simulink model "S_PIL_PVSISTEM_2026_V1"  (R2017a)
settings: Solver=VariableStepAuto  StartTime=0.0  StopTime=1.3  FixedStep=1e-6  MaxStep=1e-4  RelTol=1e-3
values from neighbouring files (symbols this model uses):
  a = 9    [M_PARAM_V1.m]    (also in M_PIL_PVSISTEM_2026_V1.m; ModTusk_V1.m)
  Alpha1 = 2*Zeta_obs*wn_obs    (= 2)    [M_PARAM_V1.m]    (also in M_PIL_PVSISTEM_2026_V1.m)
  Alpha2 = wn_obs    (= 1)    [M_PARAM_V1.m]    (also in M_PIL_PVSISTEM_2026_V1.m)
  alpha_max = 4/ts_min    (= 13333.3333333)    [M_PARAM_V1.m]    (also in M_PIL_PVSISTEM_2026_V1.m; ModTusk_V1.m)
  alpha_min = 4/ts_max    (= 259.067357513)    [M_PARAM_V1.m]    (also in M_PIL_PVSISTEM_2026_V1.m = 133.333333333; ModTusk_V1.m = 133.333333333)
  Cdc = Cdc    (= 0.0033)    [M_PARAM_V1.m]    (also in M_PIL_PVSISTEM_2026_V1.m = 0.00047)
  Cpv = Cpv    (= 0.0001)    [M_PARAM_V1.m]    (also in M_PIL_PVSISTEM_2026_V1.m = 0.0002)
  dIL = (vpv/L)*d*Ts    (= 0.46035072)    [M_PIL_PVSISTEM_2026_V1.m]
  Epsilon = Ep_cont/Ts1    [M_PARAM_V1.m]    (also in M_PIL_PVSISTEM_2026_V1.m)
  ESRCdc = ESRCdc    (= 0.2)    [M_PARAM_V1.m]    (also in M_PIL_PVSISTEM_2026_V1.m)
  ESRCpv = ESRCpv    (= 0.2)    [M_PARAM_V1.m]    (also in M_PIL_PVSISTEM_2026_V1.m)
  Fred = fs    (= 60)    [M_PARAM_V1.m]    (also in M_PIL_PVSISTEM_2026_V1.m)
  fs = 60    [M_PARAM_V1.m]    (also in M_PIL_PVSISTEM_2026_V1.m)
  Icc_calc = In/(5/100)    [M_PARAM_V1.m]    (also in M_PIL_PVSISTEM_2026_V1.m)
  K1 = Kt_acker_d    [M_PARAM_V1.m]    (also in M_PIL_PVSISTEM_2026_V1.m)
  K1y2md = Kmd(1:end-1)    [M_PARAM_V1.m]    (also in M_PIL_PVSISTEM_2026_V1.m)
  Kdpwm = 1/Ucmax    (= 0.000111111111111)    [M_PARAM_V1.m]    (also in M_PIL_PVSISTEM_2026_V1.m = 1.52590218967e-05)
  KI1 = Kp1/Ti1*Ts1    (= 760)    [M_PARAM_V1.m]    (also in M_PIL_PVSISTEM_2026_V1.m = 14.4)
  KI2 = Ki2*Ts4    [M_PARAM_V1.m]    (also in M_PIL_PVSISTEM_2026_V1.m)
  KI4 = Ki4*Ts4    [M_PARAM_V1.m]    (also in M_PIL_PVSISTEM_2026_V1.m)
  KI5 = Ki5*Ts_inv    (= 0.17765287922)    [M_PARAM_V1.m]    (also in M_PIL_PVSISTEM_2026_V1.m = 0.0710611516878)
  Kimd = -Kmd(end)    [M_PARAM_V1.m]    (also in M_PIL_PVSISTEM_2026_V1.m)
  KP1 = Kp1-KI1/2    (= 5320)    [M_PARAM_V1.m]    (also in M_PIL_PVSISTEM_2026_V1.m = 2392.8)
  KP2 = Kp2-KI2/2    [M_PARAM_V1.m]    (also in M_PIL_PVSISTEM_2026_V1.m)
  KP4 = Kp4-KI4/2    [M_PARAM_V1.m]    (also in M_PIL_PVSISTEM_2026_V1.m)
  KP5 = Kp5*Ts_inv-KI5/2    (= -0.0874937760062)    [M_PARAM_V1.m]    (also in M_PIL_PVSISTEM_2026_V1.m = -0.0349975104025)
  L = L    (= 0.0044)    [M_PARAM_V1.m]    (also in M_PIL_PVSISTEM_2026_V1.m = 0.1)
  Linv = 0.03    [M_PARAM_V1.m]    (also in M_PIL_PVSISTEM_2026_V1.m = 0.035)
  Rinv = 0.0417    [M_PARAM_V1.m]    (also in M_PIL_PVSISTEM_2026_V1.m)
  RL = RL    (= 0.494)    [M_PARAM_V1.m]    (also in M_PIL_PVSISTEM_2026_V1.m = 0.3)
  S = 10e3*3/2    (= 15000)    [M_PARAM_V1.m]    (also in M_PIL_PVSISTEM_2026_V1.m)
  Ts = Ts1    (= 0.0002)    [M_PARAM_V1.m]    (also in M_PIL_PVSISTEM_2026_V1.m)
  Ts1 = 1/Fs    (= 0.0002)    [M_PARAM_V1.m]    (also in M_PIL_PVSISTEM_2026_V1.m)
  Ts4 = 1/(4*Fc)    (= 0.000125)    [M_PARAM_V1.m]    (also in M_PIL_PVSISTEM_2026_V1.m = 5e-05)
  Ts_inv = 1/(100*Fc)    (= 5e-06)    [M_PARAM_V1.m]    (also in M_PIL_PVSISTEM_2026_V1.m = 2e-06)
  Ucmax = 9000    [M_PARAM_V1.m]    (also in M_PIL_PVSISTEM_2026_V1.m = 65535)
  vdc = 12    [M_PARAM_V1.m]    (also in M_PIL_PVSISTEM_2026_V1.m = 1000)
  vdc_ref = vdc    (= 12)    [M_PARAM_V1.m]    (also in M_PIL_PVSISTEM_2026_V1.m = 1000)
  Vf = VL/sqrt(3)    [M_PARAM_V1.m]    (also in M_PIL_PVSISTEM_2026_V1.m)
  VL = (381.051/2)    (= 190.5255)    [M_PARAM_V1.m]    (also in M_PIL_PVSISTEM_2026_V1.m)
undefined symbols (not defined in the file or in its folder): DiscIntNeverNeededParam
undefined symbols (not defined in the file): Fs
libraries: powerlib x15, powerlib_meascontrol x12, dsparch4 x3, re_lib x1
(part 2 of 2)

== matlab function S_PIL_PVSISTEM_2026_V1/Cont Real Est2/FL controller via Eq. (14) with P control law v[k] ==
  data: z_ref_k input; Kdpwm input; vdc input; L input; K1 input; u_c_k output; z_hat_k input
function u_c_k = fcn(z_ref_k, Kdpwm, vdc, L, K1, z_hat_k)
% Feedback-linearizing control law with EHGO and proportional
% auxiliary control.
%
% This controller is used as the FL-EHGO benchmark for comparison
% with the proposed FL-EHGO structure with LFA control.
%
% Inputs:
%   z_ref_k   : tracking reference z_ref[k] = i_mpp[k]
%   Kdpwm     : digital PWM gain
%   vdc       : dc-bus voltage
%   L         : boost-converter inductance
%   K1        : proportional auxiliary-control gain
%   z_hat_k   : EHGO estimates [z_hat[k]; sigma_hat[k]]
%
% Output:
%   u_c_k     : converter control input u_c[k]

% EHGO estimates
z_est_k     = z_hat_k(1);
sigma_est_k = z_hat_k(2);

% Proportional auxiliary control
v_k = -K1 * (z_est_k - z_ref_k);

% Feedback-linearizing control input according to Eq. (14)
% The nominal term b_hat is neglected in the practical implementation.
u_c_k = (L/(Kdpwm*vdc)) * ...
        (-sigma_est_k + v_k);

end

== matlab function S_PIL_PVSISTEM_2026_V1/Cont Real Est2/Look-Up Table-Based MPPT ==
  data: G input; i_mpp output; dIL input
function i_mpp = fcn(G, dIL)
% MPP current reference generation using a G-to-Impp lookup table.
%
% G       : irradiance input
% dIL     : peak-to-peak inductor-current ripple compensation
%
% Output:
% i_mpp   : compensated MPP current reference
%
% The lookup table covers G = 50...1200 W/m^2 with a 10 W/m^2 step.
% Linear interpolation is used within the table and extrapolation is
% applied outside the tabulated irradiance range.

persistent G_tab Impp_tab

if isempty(G_tab)

    G_tab = single(50:10:1200);

    Impp_tab = coder.const(double([ ...
    0.79 0.95 1.10 1.26 1.42 1.58 1.74 1.89 2.05 2.21 ...
    2.36 2.53 2.68 2.84 3.00 3.15 3.31 3.47 3.63 3.78 ...
    3.95 4.10 4.26 4.41 4.58 4.73 4.89 5.05 5.21 5.36 ...
    5.52 5.68 5.84 5.99 6.15 6.31 6.46 6.62 6.78 6.94 ...
    7.09 7.25 7.41 7.57 7.72 7.88 8.04 8.20 8.36 8.51 ...
    8.67 8.83 8.98 9.13 9.29 9.45 9.61 9.76 9.92 10.08 ...
    10.24 10.39 10.55 10.71 10.86 11.02 11.18 11.33 11.49 11.64 ...
    11.80 11.96 12.11 12.28 12.44 12.60 12.75 12.90 13.06 13.21 ...
    13.37 13.52 13.68 13.85 14.01 14.16 14.31 14.47 14.62 14.77 ...
    14.92 15.10 15.25 15.41 15.56 15.71 15.86 16.04 16.19 16.34 ...
    16.49 16.64 16.80 16.96 17.12 17.27 17.42 17.57 17.75 17.90 ...
    18.05 18.20 18.35 18.53 18.68 18.83
    ]));

end

% Nominal MPP-current interpolation
I_mpp_nom = interp1(G_tab, Impp_tab, G, 'linear', 'extrap');

% Inductor-current ripple compensation
i_mpp = I_mpp_nom - dIL;

% Prevent negative current-reference values
i_mpp = max(i_mpp, 0);

end

== matlab function S_PIL_PVSISTEM_2026_V1/Cont Real Est1/PID Digital I 3 ==
  data: x1k_ref input; uck output; x1k input; KI input; KP input
function uck = fcn(x1k_ref, x1k, KI, KP)
% Discrete-time PI controller used as a benchmark MPPT controller.
%
% Inputs:
%   x1k_ref : current reference at sampling instant k
%   x1k     : measured current at sampling instant k
%   KI      : discrete integral gain
%   KP      : proportional gain
%
% Output:
%   uck     : control signal at sampling instant k

% Persistent variables used to store the current and previous
% error and control-signal values
persistent ek uk
persistent ek_1 uk_1

% Initialize persistent variables at the beginning of the simulation
if isempty(ek)
    ek = 0;
    uk = 0;
    ek_1 = 0;
    uk_1 = 0;
end

% Tracking error
ek = x1k_ref - x1k;

% Incremental discrete-time PI control law
uk = ek*(KP + KI) - ek_1*KP + uk_1;

% Store current values for the next sampling instant
ek_1 = ek;
uk_1 = uk;

% Controller output
uck = uk;

end

== matlab function S_PIL_PVSISTEM_2026_V1/Measurements 2/Subsystem3/MATLAB Function ==
  data: uc_avg output; uc input; time input; t_start input; t_end input
function uc_avg = control_effort_avg(uc, time, t_start, t_end)
%#codegen
% Calcula el valor promedio acumulado del esfuerzo de control
% solo dentro del intervalo [t_start, t_end].
%
% Entradas:
%   uc      : señal de control instantánea (ej. ciclo de trabajo o voltaje)
%   time    : tiempo actual (segundos)
%   t_start : tiempo desde el cual se comienza a acumular
%   t_end   : tiempo en el que se detiene la acumulación
%
% Salida:
%   uc_avg : valor promedio acumulado del esfuerzo de control

% Variables persistentes
persistent sum_u sample_count started

% Inicialización
if isempty(sum_u)
    sum_u = 0;
    sample_count = 0;
    started = false;
end

% Acumulación solo dentro del intervalo [t_start, t_end]
if time >= t_start && time <= t_end
    if ~started
        started = true; % se activa solo la primera vez que entra al intervalo
    end

    sum_u = sum_u + abs(uc); % acumulación del valor absoluto
    sample_count = sample_count + 1;
end

% Cálculo del promedio acumulado
if sample_count == 0
    uc_avg = 0;
else
    uc_avg = sum_u / sample_count;
end
end

== matlab function S_PIL_PVSISTEM_2026_V1/Cont Real Est5/Look-Up Table-Based MPPT ==
  data: G input; i_mpp output; dIL input
function i_mpp = fcn(G, dIL)
% MPP current reference generation using a G-to-Impp lookup table.
%
% G       : irradiance input
% dIL     : peak-to-peak inductor-current ripple compensation
%
% Output:
% i_mpp   : compensated MPP current reference
%
% The lookup table covers G = 50...1200 W/m^2 with a 10 W/m^2 step.
% Linear interpolation is used within the table and extrapolation is
% applied outside the tabulated irradiance range.

persistent G_tab Impp_tab

if isempty(G_tab)

    G_tab = single(50:10:1200);

    Impp_tab = coder.const(double([ ...
    0.79 0.95 1.10 1.26 1.42 1.58 1.74 1.89 2.05 2.21 ...
    2.36 2.53 2.68 2.84 3.00 3.15 3.31 3.47 3.63 3.78 ...
    3.95 4.10 4.26 4.41 4.58 4.73 4.89 5.05 5.21 5.36 ...
    5.52 5.68 5.84 5.99 6.15 6.31 6.46 6.62 6.78 6.94 ...
    7.09 7.25 7.41 7.57 7.72 7.88 8.04 8.20 8.36 8.51 ...
    8.67 8.83 8.98 9.13 9.29 9.45 9.61 9.76 9.92 10.08 ...
    10.24 10.39 10.55 10.71 10.86 11.02 11.18 11.33 11.49 11.64 ...
    11.80 11.96 12.11 12.28 12.44 12.60 12.75 12.90 13.06 13.21 ...
    13.37 13.52 13.68 13.85 14.01 14.16 14.31 14.47 14.62 14.77 ...
    14.92 15.10 15.25 15.41 15.56 15.71 15.86 16.04 16.19 16.34 ...
    16.49 16.64 16.80 16.96 17.12 17.27 17.42 17.57 17.75 17.90 ...
    18.05 18.20 18.35 18.53 18.68 18.83
    ]));

end

% Nominal MPP-current interpolation
I_mpp_nom = interp1(G_tab, Impp_tab, G, 'linear', 'extrap');

% Inductor-current ripple compensation
i_mpp = I_mpp_nom - dIL;

% Prevent negative current-reference values
i_mpp = max(i_mpp, 0);

end

== matlab function S_PIL_PVSISTEM_2026_V1/Measurements 2/Subsystem6/MATLAB Function ==
  data: ah output; current input; time input; t_start input; t_end input; i_avg output
function [ah, i_avg] = ah_accumulator(current, time, t_start, t_end)
%#codegen
% Calcula la carga acumulada en Ah y la corriente promedio en el intervalo [t_start, t_end]

% Entradas:
%   current : corriente instantánea (A)
%   time    : tiempo actual (s)
%   t_start : tiempo de inicio del intervalo (s)
%   t_end   : tiempo de fin del intervalo (s)
%
% Salidas:
%   ah    : carga acumulada en Ah
%   i_avg : corriente promedio (A)

% Variables persistentes
persistent last_time total_Ah started current_sum sample_count

% Inicialización al primer uso
if isempty(total_Ah)
    total_Ah = 0;
    last_time = 0;
    started = false;
    current_sum = 0;
    sample_count = 0;
end

% Solo acumular si dentro del intervalo
if time >= t_start && time <= t_end
    if ~started
        last_time = time;
        started = true;
    end

    dt = time - last_time;
    if dt > 0
        total_Ah = total_Ah + (current * dt) / 3600;
        last_time = time;
    end

    % Acumular para promedio
    current_sum = current_sum + current;
    sample_count = sample_count + 1;
end

% Resultados
ah = total_Ah;

% Corriente promedio solo si hay muestras válidas
if sample_count > 0
    i_avg = current_sum / sample_count;
else
    i_avg = 0;
end
end

== matlab function S_PIL_PVSISTEM_2026_V1/Cont Real Est3/EHGO via Eq. (13) ==
  data: y_k input; alpha_1 input; alpha_2 input; epsilon input; Kdpwm input; vdc input; L input; Ts input; u_c_k input; z_hat_k input; z_hat_next output
function z_hat_next = fcn(y_k, alpha_1, alpha_2, epsilon, ...
                          Kdpwm, vdc, L, Ts, u_c_k, z_hat_k)
% Discrete-time extended high-gain observer (EHGO).
%
% Inputs:
%   y_k       : measured output y[k]
%   alpha_1   : first EHGO coefficient
%   alpha_2   : second EHGO coefficient
%   epsilon   : high-gain observer tuning parameter
%   Kdpwm     : DPWM gain
%   vdc       : dc-bus voltage
%   L         : Boost-converter inductance
%   Ts        : sampling period
%   u_c_k     : converter control input u_c[k]
%   z_hat_k   : current EHGO state estimates
%
% Output:
%   z_hat_next : EHGO state estimates at k+1

z_hat_next = zeros(2,1);

% Output-estimation error
e_obs_k = y_k - z_hat_k(1);

% EHGO state update
z_hat_next(1) = z_hat_k(1) + Ts * ( ...
    z_hat_k(2) + ...
    ((Kdpwm/L)*vdc)*u_c_k + ...
    (alpha_1/(epsilon*Ts))*e_obs_k );

z_hat_next(2) = z_hat_k(2) + Ts * ( ...
    (alpha_2/(epsilon^2*Ts^2))*e_obs_k );

end

== matlab function S_PIL_PVSISTEM_2026_V1/Cont Real Est3/Feedback-linearizing control via Eq. (14) ==
  data: Kdpwm input; vdc input; L input; v_k input; u_c_k output; z_hat_2_k input
function u_c_k = fcn(Kdpwm, vdc, L, v_k, z_hat_2_k)
% Feedback-linearizing control law using the EHGO estimate.
%
% Inputs:
%   Kdpwm       : DPWM gain
%   vdc         : dc-bus voltage
%   L           : Boost-converter inductance
%   v_k         : LFA auxiliary control v[k]
%   z_hat_2_k   : second EHGO state estimate
%
% Output:
%   u_c_k       : converter control input u_c[k]

u_c_k = (L/(Kdpwm*vdc)) * ...
        (-z_hat_2_k + v_k);

end

== matlab function S_PIL_PVSISTEM_2026_V1/Cont Real Est3/LUT-based MPPT ==
  data: G_k input; I_mpp_k output; dIL_k input
function I_mpp_k = fcn(G_k, dIL_k)
% MPP current reference generation using a G-to-Impp lookup table.
%
% G       : irradiance input
% dIL     : peak-to-peak inductor-current ripple compensation
%
% Output:
% i_mpp   : compensated MPP current reference
%
% The lookup table covers G = 50...1200 W/m^2 with a 10 W/m^2 step.
% Linear interpolation is used within the table and extrapolation is
% applied outside the tabulated irradiance range.

persistent G_tab Impp_tab

if isempty(G_tab)

    G_tab = single(50:10:1200);

    Impp_tab = coder.const(double([ ...
    0.79 0.95 1.10 1.26 1.42 1.58 1.74 1.89 2.05 2.21 ...
    2.36 2.53 2.68 2.84 3.00 3.15 3.31 3.47 3.63 3.78 ...
    3.95 4.10 4.26 4.41 4.58 4.73 4.89 5.05 5.21 5.36 ...
    5.52 5.68 5.84 5.99 6.15 6.31 6.46 6.62 6.78 6.94 ...
    7.09 7.25 7.41 7.57 7.72 7.88 8.04 8.20 8.36 8.51 ...
    8.67 8.83 8.98 9.13 9.29 9.45 9.61 9.76 9.92 10.08 ...
    10.24 10.39 10.55 10.71 10.86 11.02 11.18 11.33 11.49 11.64 ...
    11.80 11.96 12.11 12.28 12.44 12.60 12.75 12.90 13.06 13.21 ...
    13.37 13.52 13.68 13.85 14.01 14.16 14.31 14.47 14.62 14.77 ...
    14.92 15.10 15.25 15.41 15.56 15.71 15.86 16.04 16.19 16.34 ...
    16.49 16.64 16.80 16.96 17.12 17.27 17.42 17.57 17.75 17.90 ...
    18.05 18.20 18.35 18.53 18.68 18.83
    ]));

end

% Nominal MPP-current interpolation
I_mpp_nom = interp1(G_tab, Impp_tab, G_k, 'linear', 'extrap');

% Inductor-current ripple compensation
I_mpp_k = I_mpp_nom - dIL_k;

% Prevent negative current-reference values
I_mpp_k = max(I_mpp_k, 0);

end

== matlab function S_PIL_PVSISTEM_2026_V1/Cont Real Est5/PID Digital I 2 ==
  data: x1k_Ref input; x1k input; x2k input; uck output; Ki input; K1 input; K2 input; Ts input
function uck = fcn(x1k_Ref, x1k, x2k, Ki, K1, K2, Ts)
% State-feedback controller with integral action used as a benchmark
% MPPT controller.
%
% Inputs:
%   x1k_Ref : current reference at sampling instant k
%   x1k     : first measured state at sampling instant k
%   x2k     : second measured state at sampling instant k
%   Ki      : integral gain
%   K1      : state-feedback gain associated with x1k
%   K2      : state-feedback gain associated with x2k
%   Ts      : sampling period
%
% Output:
%   uck     : control signal at sampling instant k

% Persistent variables used to preserve the controller states
% between consecutive sampling instants
persistent ek Acc_Int Acc_Int_1 uk

% Initialize persistent variables at the beginning of the simulation
if isempty(ek)
    ek = 0;
    Acc_Int = 0;
    Acc_Int_1 = 0;
    uk = 0;
end

% Tracking error
ek = x1k_Ref - x1k;

% Discrete-time integral action
Acc_Int = Ki * ek * Ts + Acc_Int_1;
Acc_Int_1 = Acc_Int;

% Control law: integral action combined with state feedback
uk = Acc_Int - (K1 * x1k + K2 * x2k);

% Controller output
uck = uk;

end

== matlab function S_PIL_PVSISTEM_2026_V1/Measurements 2/Subsystem12/MATLAB Function ==
  data: efficiency output; Pmpp input; Pactual input; time input; t_start input; t_end input

function efficiency = n_mppt(Pmpp, Pactual, time, t_start, t_end)
%#codegen
% Calcula la eficiencia acumulada de un MPPT en porcentaje
% limitando Pactual para que no exceda Pmpp.
% Acumula solo dentro del intervalo de tiempo [t_start, t_end].
%
% Entradas:
%   Pmpp     : potencia teórica máxima (kW)
%   Pactual  : potencia medida real (kW)
%   time     : tiempo actual (segundos)
%   t_start  : inicio de acumulación
%   t_end    : fin de acumulación
%
% Salida:
%   efficiency : eficiencia acumulada (%), limitada a 100

% Variables persistentes
persistent total_Pmpp total_Pactual started

% Inicialización al primer uso
if isempty(total_Pmpp)
    total_Pmpp = 0;
    total_Pactual = 0;
    started = false;
end

% Acumular solo dentro del intervalo [t_start, t_end]
if time >= t_start && time <= t_end
    if ~started
        started = true;
    end

    % Limitar Pactual para evitar que exceda Pmpp
    %Pactual_limited = min(Pactual, Pmpp);
     
    % No Limitar Pactual 
    Pactual_limited = Pactual;

    % Acumulación
    total_Pmpp = total_Pmpp + Pmpp;
    total_Pactual = total_Pactual + Pactual_limited;
end

% Cálculo de eficiencia acumulada
if total_Pmpp < 1e-6
    efficiency = 0;
else
    efficiency = min((total_Pactual / total_Pmpp) * 100, 100);
end
end

== matlab function S_PIL_PVSISTEM_2026_V1/Cont Real Est3/PID Digital I 3 ==
  data: alpha_k input; z_ref_k input; Ts input; v_k output; z_k input
function v_k = fcn(alpha_k, z_ref_k, Ts, z_k)
% LFA auxiliary control implementation.
%
% The decay rate alpha[k], provided by the two-rule Tsukamoto fuzzy
% inference system, determines the discrete-time contraction factor
% lambda[k]. The adaptive gains K[k] and L[k] are then computed to
% generate the auxiliary control v[k].
%
% Inputs:
%   alpha_k : Decay rate alpha[k] provided by the fuzzy inference system
%   z_ref_k : Tracking reference z_ref[k] = i_mpp[k]
%   Ts      : Sampling period
%   z_k     : Feedback-linearized state z[k]
%
% Output:
%   v_k     : Auxiliary control v[k]

% Numerical protection
alpha_k = max(alpha_k, eps);

% Contraction factor - equation (35)
lambda_k = exp(-alpha_k * Ts);

% Adaptive auxiliary-control gains - equation (34)
K_k = (1 - lambda_k) / Ts;
L_k = (1 - lambda_k) / Ts;

% LFA auxiliary control law - equation (34)
v_k = -K_k * z_k + L_k * z_ref_k;

end

== matlab function S_PIL_PVSISTEM_2026_V1/Measurements 2/Subsystem14/MATLAB Function ==
  data: energy_wh output; power_kw input; time input; t_start input; t_end input; power_avg output
function [energy_wh, power_avg] = wh_accumulator(power_kw, time, t_start, t_end)
%#codegen
% Calcula la energía acumulada (Wh) y potencia promedio (kW)
% dentro del intervalo de tiempo [t_start, t_end].

% Entradas:
%   power_kw : potencia instantánea en kilowatts (kW)
%   time     : tiempo actual (s)
%   t_start  : tiempo inicial (s)
%   t_end    : tiempo final (s)
%
% Salidas:
%   energy_wh : energía acumulada en Wh
%   power_avg : potencia promedio en kW

% Variables persistentes
persistent last_time total_energy_wh started sum_power sample_count

% Inicialización al primer uso
if isempty(total_energy_wh)
    total_energy_wh = 0;
    last_time = 0;
    started = false;
    sum_power = 0;
    sample_count = 0;
end

% Solo acumular si dentro del intervalo
if time >= t_start && time <= t_end
    if ~started
        last_time = time;
        started = true;
    end

    dt = time - last_time;
    if dt > 0
        % Energía en Wh: P(kW) * dt (s) * (1000 / 3600)
        total_energy_wh = total_energy_wh + (power_kw * dt) * (1000 / 3600);
        last_time = time;
    end

    % Para el promedio de potencia
    sum_power = sum_power + power_kw;
    sample_count = sample_count + 1;
end

% Salidas
energy_wh = total_energy_wh;

if sample_count > 0
    power_avg = 1000*(sum_power / sample_count);
else
    power_avg = 0;
end
end

== matlab function S_PIL_PVSISTEM_2026_V1/Cont Real Est3/Tsukamoto General1 ==
  data: a input; alpha_min input; alpha_max input; ek input; alpha_k output
function alpha_k = fcn(a, alpha_min, alpha_max, ek)
% General two-rule Tsukamoto implementation with w1 = exp(...)
%
% ek         : tracking error (scalar or vector)
% a          : Gaussian width parameter for mu_A1(|ek|)
% alpha_min  : lower bound of the physical decay-rate interval
% alpha_max  : upper bound of the physical decay-rate interval
%
% Output:
% alpha_k    : decay rate alpha[k] in [alpha_min, alpha_max]

% Numerical protection
a = max(a, eps);

% Width of the physical decay-rate interval
Delta_alpha = alpha_max - alpha_min;

% Centered output universe
alpha_c_min = -Delta_alpha/2;
alpha_c_max =  Delta_alpha/2;

% Input fuzzification based on the tracking-error magnitude
e_abs = abs(ek);

w1 = exp(-(e_abs.^2)/(2*a^2));   % mu_A1(|ek|): small tracking error
w2 = 1 - w1;                     % mu_A2(|ek|): large tracking error

% Tsukamoto inversion for alpha_c in
% [alpha_c_min, alpha_c_max]
z1 = alpha_c_max - w1.*Delta_alpha;  % R1: A1 -> B2 (decreasing)
z2 = alpha_c_min + w2.*Delta_alpha;  % R2: A2 -> B1 (increasing)

% Normalized weighted aggregation in the centered universe
den = w1 + w2;
den(den < eps) = eps;

alpha_c = ...
    (w1.*z1 + w2.*z2) ./ den;

% Translation to the physical decay-rate interval
alpha_k = ...
    alpha_c + ...
    (alpha_min + alpha_max)/2;

% Optional numerical saturation
alpha_k = ...
    min(max(alpha_k, alpha_min), alpha_max);

end
